simulink library "syntheticFlow_ul"  (R2022a)
settings: Solver=VariableStepAuto  StartTime=0.0  StopTime=10.0  RelTol=1e-3
undefined symbols (not defined in the file or in its folder): tt
libraries: simulink x1
settings Model: Creator=Ayaz  LastModifiedBy=lhill8
settings SolverCC: AlgebraicLoopSolver=TrustRegion
settings DebuggingCC: UnconnectedInputMsg=warning  UnconnectedOutputMsg=warning  UnconnectedLineMsg=warning  SFMachineParentedDataDiag=warning

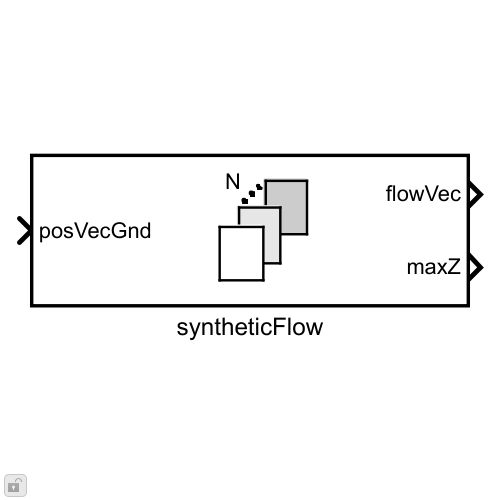
[thumbnail: Simulink's stored preview of the top-level diagram]
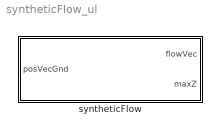
== system syntheticFlow_ul ==
  syntheticFlow : Subsystem  mask{en=tt}
      mask prompts: en "Environment object"
      mask init:
      | [synFlow,zVals] = en.water.generateData();

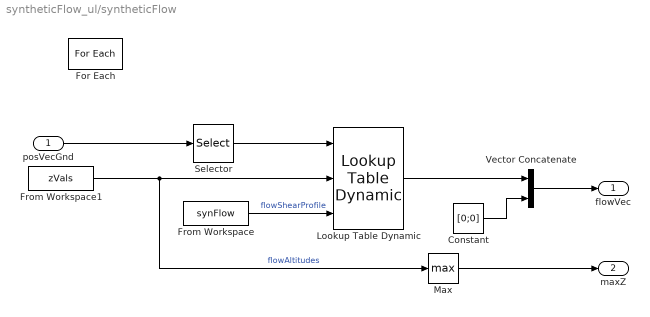
== system syntheticFlow_ul/syntheticFlow ==
  posVecGnd : Inport  Partition=on  PartitionDimension=2  PartitionWidth=1  PartitionOffset=0
  Constant : Constant  Value=[0;0]  VectorParams1D=off
  For Each : ForEach  DisableCoverage=on
  From Workspace : FromWorkspace  VariableName=synFlow
  From Workspace1 : FromWorkspace  VariableName=zVals
  Lookup Table Dynamic : simulink/Lookup Tables/Lookup Table Dynamic  LookUpMeth=Interpolation-Use End Values  OutDataType=fixdt('double')  OutScaling=[]  OutputDataTypeScalingMode=Specify via dialog  OutDataTypeStr=double  DoSatur=off
  Max : MinMax  Function=max
  Selector : Selector  InputPortWidth=3  IndexOptions=Index vector (dialog)  Indices=[3]  OutputSizes=1
  Vector Concatenate : Concatenate
  flowVec : Outport  PortDimensions=[3;1]  ConcatenationDimension=2
  maxZ : Outport  Port=2  ConcatenationDimension=1
  wires:
  From Workspace/1 -> Lookup Table Dynamic/3  "flowShearProfile"
  From Workspace1/1 -> Lookup Table Dynamic/2, Max/1  "flowAltitudes"
  posVecGnd/1 -> Selector/1
  Lookup Table Dynamic/1 -> Vector Concatenate/1
  Max/1 -> maxZ/1
  Selector/1 -> Lookup Table Dynamic/1
  Constant/1 -> Vector Concatenate/2
  Vector Concatenate/1 -> flowVec/1
